simulink library "emergency_stop_algorithm_atomic_sub_chart_library"  (R2013a)
settings: Solver=ode45  StartTime=0.0  StopTime=10.0  RelTol=1e-3
settings Model: Creator=mbiesiad  LastModifiedBy=mbiesiad

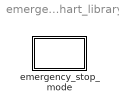
== system emergency_stop_algorithm_atomic_sub_chart_library ==
  emergency_stop_mode : Stateflow chart  TreatAsAtomicUnit=on

== stateflow chart emergency_stop_algorithm_atomic_sub_chart_library/emergency_stop_mode ==
  state emergency_stop
    during:
